simulink model "activemodel01"  (R2025b)
settings: Solver=VariableStepAuto  StartTime=0.0  StopTime=10  RelTol=1e-3
libraries: simulink x1
settings Model: Creator=claygrant  LastModifiedBy=wangxuanyi

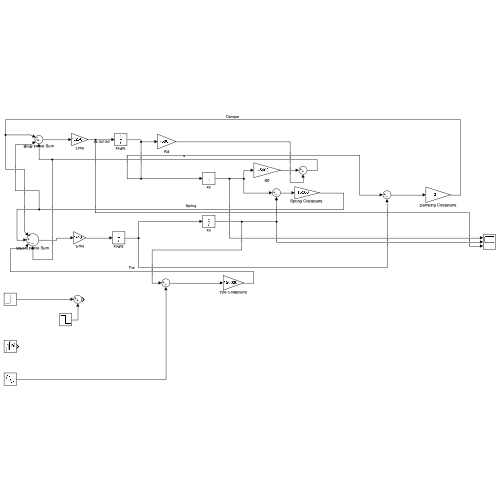
[thumbnail: Simulink's stored preview of the top-level diagram]
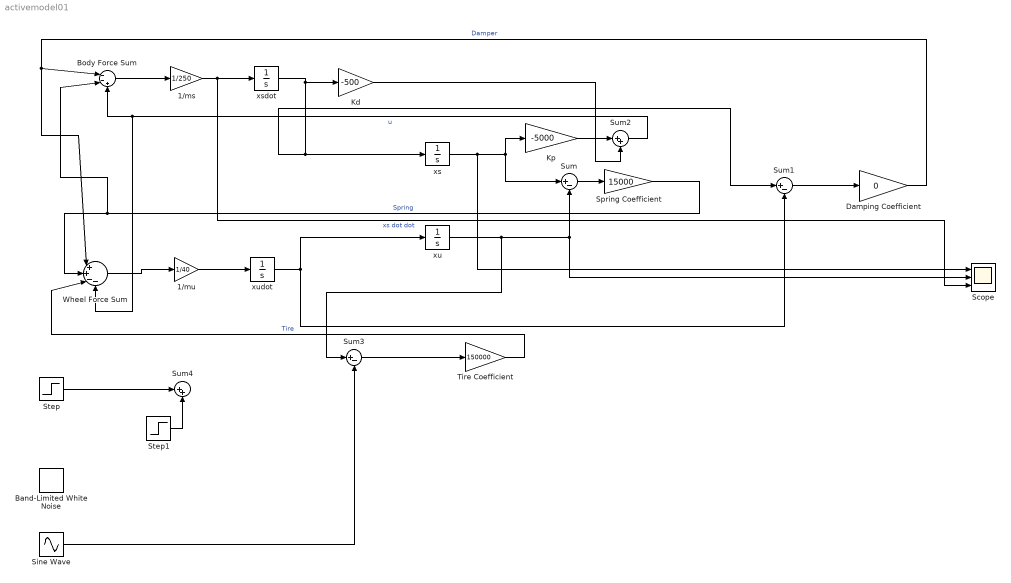
== system activemodel01 ==
  1/ms : Gain  Gain=1/250
  1/mu : Gain  Gain=1/40
  Band-Limited White Noise : simulink/Sources/Band-Limited White Noise  Cov=[1e-4]  Ts=1  seed=[23341]
  Body Force Sum : Sum  Inputs=|--+
  Damping Coefficient : Gain  Gain=0
  Kd : Gain  Gain=-500
  Kp : Gain  Gain=-5000
  Scope : Scope  NumInputPorts=3
      settings: ActiveDisplayYMinimum=-0.057257543771014496  ActiveDisplayYMaximum=0.10959310601453244
  Sine Wave : Sin  Amplitude=0.02  Frequency=10  SampleTime=0
  "Spring Coefficient " : Gain  Gain=15000
  Step : Step  After=0.05  SampleTime=0
  Step1 : Step  Time=1.5  After=-0.05  SampleTime=0
  Sum : Sum  Inputs=|+-
  Sum1 : Sum  Inputs=|+-
  Sum2 : Sum  Inputs=|++
  Sum3 : Sum  Inputs=|+-
  Sum4 : Sum  Inputs=|++
  Tire Coefficient : Gain  Gain=150000
  Wheel Force Sum : Sum  Inputs=|++--
  xs : Integrator
  xsdot : Integrator
  xu : Integrator
  xudot : Integrator
  wires:
  xu/1 -> Sum3/1, Scope/2, Sum/2
  Sum/1 -> "Spring Coefficient "/1
  xsdot/1 -> Kd/1, Sum1/1, xs/1
  xudot/1 -> xu/1, Sum1/2
  Sum1/1 -> Damping Coefficient/1
  Wheel Force Sum/1 -> 1/mu/1
  Body Force Sum/1 -> 1/ms/1
  1/ms/1 -> Scope/3, xsdot/1  "xs dot dot"
  1/mu/1 -> xudot/1
  "Spring Coefficient "/1 -> Wheel Force Sum/2, Body Force Sum/2  "Spring"
  Damping Coefficient/1 -> Wheel Force Sum/1, Body Force Sum/1  "Damper"
  Sum3/1 -> Tire Coefficient/1
  Tire Coefficient/1 -> Wheel Force Sum/3  "Tire"
  xs/1 -> Scope/1, Sum/1, Kp/1
  Kp/1 -> Sum2/1
  Kd/1 -> Sum2/2
  Sum2/1 -> Wheel Force Sum/4, Body Force Sum/3  "u"
  Step/1 -> Sum4/1
  Step1/1 -> Sum4/2
  Sine Wave/1 -> Sum3/2
